simulink model "quad_control_loops"  (R2026a)
settings: Solver=ode45  StopTime=25
InitFcn:
  | setup_control
values from neighbouring files (symbols this model uses):
  A_aug = [A9, zeros(9,1); zeros(1,8), -1, 0]    [setup_control.m]
  B_aug = [B9; zeros(1,4)]    [setup_control.m]
  C_aug = eye(10)    [setup_control.m]
  D_aug = zeros(10,4)    [setup_control.m]
  K =     [control_gains.mat]    (also in setup_control.m = G.K; sim_control_compare.m = G.K; sim_control_linear.m = G.K; sim_control_nonlinear.m = G.K)
  X0_aug = zeros(10,1)    [setup_control.m]
settings Model: Creator=graest  LastModifiedBy=graest

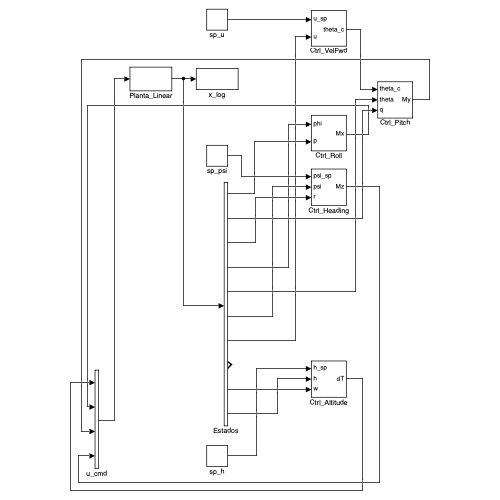
[thumbnail: Simulink's stored preview of the top-level diagram]
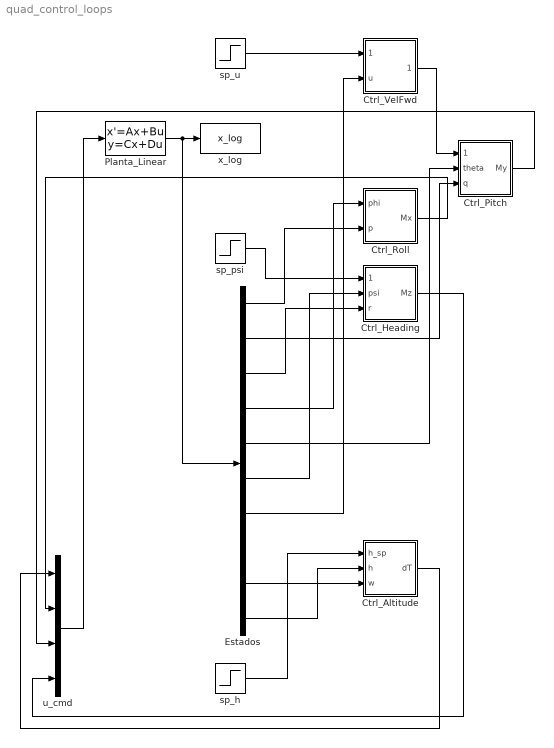
== system quad_control_loops ==
  Ctrl_Altitude : Subsystem
  Ctrl_Heading : Subsystem
  Ctrl_Pitch : Subsystem
  Ctrl_Roll : Subsystem
  Ctrl_VelFwd : Subsystem
  Estados : Demux  Outputs=10
  Planta_Linear : StateSpace  A=A_aug  B=B_aug  C=C_aug  D=D_aug  InitialCondition=X0_aug
  sp_h : Step  FinalValue=2  SampleTime=0
  sp_psi : Step  Time=16  FinalValue=0.5236  SampleTime=0
  sp_u : Step  Time=8  FinalValue=3  SampleTime=0
  u_cmd : Mux
  x_log : ToWorkspace  VariableName=x_log  SaveFormat=Timeseries  SampleTime=-1
  wires:
  Ctrl_Pitch/1(My) -> u_cmd/3
  Ctrl_VelFwd/1(theta_c) -> Ctrl_Pitch/1(theta_c)
  sp_h/1 -> Ctrl_Altitude/1(h_sp)
  Estados/10 -> Ctrl_Altitude/2(h)
  Estados/9 -> Ctrl_Altitude/3(w)
  Ctrl_Roll/1(Mx) -> u_cmd/2
  Estados/3 -> Ctrl_Heading/3(r)
  Estados/2 -> Ctrl_Pitch/3(q)
  Estados/6 -> Ctrl_Heading/2(psi)
  Ctrl_Heading/1(Mz) -> u_cmd/4
  Estados/1 -> Ctrl_Roll/2(p)
  Estados/5 -> Ctrl_Pitch/2(theta)
  sp_u/1 -> Ctrl_VelFwd/1(u_sp)
  Estados/4 -> Ctrl_Roll/1(phi)
  Ctrl_Altitude/1(dT) -> u_cmd/1
  u_cmd/1 -> Planta_Linear/1
  Planta_Linear/1 -> x_log/1, Estados/1
  Estados/7 -> Ctrl_VelFwd/2(u)
  sp_psi/1 -> Ctrl_Heading/1(psi_sp)

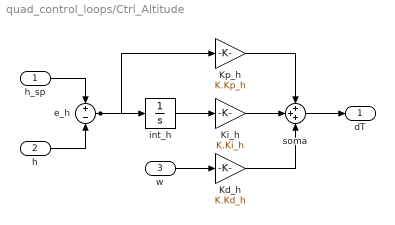
== system quad_control_loops/Ctrl_Altitude ==
  h_sp : Inport
  h : Inport  Port=2
  w : Inport  Port=3
  Kd_h : Gain  Gain=K.Kd_h
  Ki_h : Gain  Gain=K.Ki_h
  Kp_h : Gain  Gain=K.Kp_h
  e_h : Sum  Inputs=+-
  int_h : Integrator  LimitOutput=on  UpperSaturationLimit=5  LowerSaturationLimit=-5
  soma : Sum  Inputs=+++
  dT : Outport
  wires:
  soma/1 -> dT/1
  Kd_h/1 -> soma/3
  Kp_h/1 -> soma/1
  Ki_h/1 -> soma/2
  w/1 -> Kd_h/1
  e_h/1 -> int_h/1, Kp_h/1
  h/1 -> e_h/2
  int_h/1 -> Ki_h/1
  h_sp/1 -> e_h/1

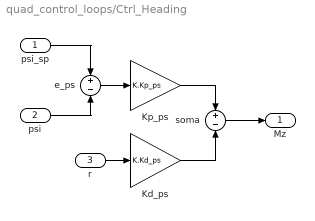
== system quad_control_loops/Ctrl_Heading ==
  psi_sp : Inport
  psi : Inport  Port=2
  r : Inport  Port=3
  Kd_ps : Gain  Gain=K.Kd_ps
  Kp_ps : Gain  Gain=K.Kp_ps
  e_ps : Sum  Inputs=+-
  soma : Sum  Inputs=+-
  Mz : Outport
  wires:
  Kd_ps/1 -> soma/2
  Kp_ps/1 -> soma/1
  r/1 -> Kd_ps/1
  soma/1 -> Mz/1
  e_ps/1 -> Kp_ps/1
  psi/1 -> e_ps/2
  psi_sp/1 -> e_ps/1

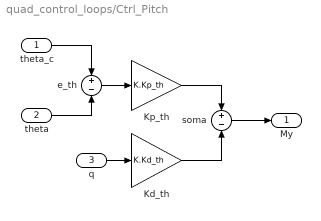
== system quad_control_loops/Ctrl_Pitch ==
  theta_c : Inport
  theta : Inport  Port=2
  q : Inport  Port=3
  Kd_th : Gain  Gain=K.Kd_th
  Kp_th : Gain  Gain=K.Kp_th
  e_th : Sum  Inputs=+-
  soma : Sum  Inputs=+-
  My : Outport
  wires:
  Kd_th/1 -> soma/2
  q/1 -> Kd_th/1
  Kp_th/1 -> soma/1
  e_th/1 -> Kp_th/1
  soma/1 -> My/1
  theta/1 -> e_th/2
  theta_c/1 -> e_th/1

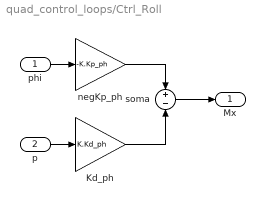
== system quad_control_loops/Ctrl_Roll ==
  phi : Inport
  p : Inport  Port=2
  Kd_ph : Gain  Gain=K.Kd_ph
  negKp_ph : Gain  Gain=-K.Kp_ph
  soma : Sum  Inputs=+-
  Mx : Outport
  wires:
  Kd_ph/1 -> soma/2
  soma/1 -> Mx/1
  negKp_ph/1 -> soma/1
  p/1 -> Kd_ph/1
  phi/1 -> negKp_ph/1

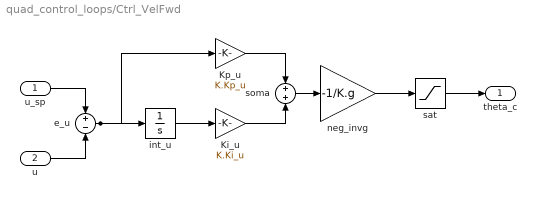
== system quad_control_loops/Ctrl_VelFwd ==
  u_sp : Inport
  u : Inport  Port=2
  Ki_u : Gain  Gain=K.Ki_u
  Kp_u : Gain  Gain=K.Kp_u
  e_u : Sum  Inputs=+-
  int_u : Integrator  LimitOutput=on  UpperSaturationLimit=5  LowerSaturationLimit=-5
  neg_invg : Gain  Gain=-1/K.g
  sat : Saturate  UpperLimit=0.34907  LowerLimit=-0.34907
  soma : Sum
  theta_c : Outport
  wires:
  sat/1 -> theta_c/1
  soma/1 -> neg_invg/1
  e_u/1 -> int_u/1, Kp_u/1
  Kp_u/1 -> soma/1
  neg_invg/1 -> sat/1
  int_u/1 -> Ki_u/1
  Ki_u/1 -> soma/2
  u/1 -> e_u/2
  u_sp/1 -> e_u/1
